simulink model "TestSFC_org"  (Simulink 10.0)
settings: Solver=ode45  StartTime=0.0  StopTime=10.0  RelTol=1e-3  EnableMultiTasking=on
libraries: Lib_Turbo_SFCCalc_TMATS x1
settings Model: Creator=tlavelle  LastModifiedBy=annonymous
settings DataIOCC: LimitDataPoints=on
settings OptimizationCC: ExpressionDepthLimit=2147483647
settings DebuggingCC: SolverPrmCheckMsg=warning  StateNameClashWarn=warning
settings GRTTargetCC: GeneratePreprocessorConditionals=Disable all  CombineOutputUpdateFcns=on  GRTInterface=off
settings ConfigComp: CovExternalEMLEnable=off

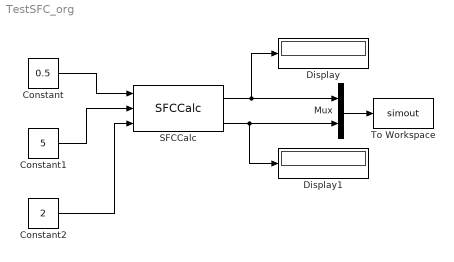
== system TestSFC_org ==
  Constant : Constant  Value=0.5
  Constant1 : Constant  Value=5
  Constant2 : Constant  Value=2
  Display : Display
  Display1 : Display
  Mux : Mux  Inputs=2
  SFCCalc : Lib_Turbo_SFCCalc_TMATS/SFCCalc
  To Workspace : ToWorkspace  VariableName=simout  SaveFormat=Timeseries  SampleTime=-1
  wires:
  SFCCalc/1 -> Display/1, Mux/1
  SFCCalc/2 -> Display1/1, Mux/2
  Mux/1 -> To Workspace/1
  Constant/1 -> SFCCalc/1
  Constant1/1 -> SFCCalc/2
  Constant2/1 -> SFCCalc/3
